simulink model "Vehicle14DOFSystemRack"  (R2024a)
settings: Solver=ode4  StartTime=0.0  StopTime=100  FixedStep=0.001  RelTol=1e-3
values from neighbouring files (symbols this model uses):
  EnvGrvty = 9.81    [Par.m]
  PlntBattChrgMax = 4.493    [Par.m]
  PlntBattNumCellSer = 96    [Par.m]
  PlntBattOpenCirctVolt = [3.17242 3.17242 3.17242 3.17242 3.17242 3.17242 3.17242;3.18272 3.18272 3.18272 3.18272 3.18272 3.18272 3.18272;3.19302 3.19302 3.19302 3.19302 3.19302 3.19302 3.19302;3.20331 3.20331 3.20331 3.20331 3.20331 3.20331 3.20331;3.21361 3.21361 3.21361 3.21361 3.21361 3.21361 3.21361;3.22391 3.22391 3.22391 3.22391 3.22391 3.22391 3.22391;3.23421 3.23421 3.23421 3.23421 3.23421 3.23421 3.23421;3.24451 ...(+5187 chars)    [Par.m]
  PlntBattSocInit = 0.6    [Par.m]
  PlntBattTempBpt = [-40 -30 -20 0 23 45 60]    [Par.m]
  PlntBattTempInitDegC = 25    [Par.m]
  PlntBattVoltSocBpt = [0 0.01 0.02 0.03 0.04 0.05 0.06 0.07 0.08 0.09 0.1 0.11 0.12 0.13 0.14 0.15 0.16 0.17 0.18 0.19 0.2 0.21 0.22 0.23 0.24 0.25 0.26 0.27 0.28 0.29 0.3 0.31 0.32 0.33 0.34 0.35 0.36 0.37 0.38 0.39 0.4 0.41 0.42 0.43 0.44 0.45 0.46 0.47 0.48 0.49 0.5 0.51 0.52 0.53 0.54 0.55 0.56 0.57 0.58 0.59 0.6 0.61 0.62 0.63 0.64 0.65 0.66 0.67 0.68 0.69 0.7 0.71 0.72 0.73 0.74 0.75 0.76 0.77 0.78 0.79 0.8 0.81  ...(+91 chars)    [Par.m]
  PlntDCDCVoltInit = 650    [Par.m]
  PlntDriveshftDamp = 100    [Par.m]
  PlntDriveshftStiff = 500    [Par.m]
  PlntEM1RotDamp = 0.001    [Par.m]
  PlntEM1RotInertia = 0.01    [Par.m]
  PlntEM2RotDamp = 0.001    [Par.m]
  PlntEM2RotInertia = 0.01    [Par.m]
  PlntEM3RotDamp = 0.001    [Par.m]
  PlntEM3RotInertia = 0.01    [Par.m]
  PlntEM4RotDamp = 0.001    [Par.m]
  PlntEM4RotInertia = 0.01    [Par.m]
  PlntEMWhlGearRatioFL = 11.04    [Par.m]
  PlntEMWhlGearRatioFR = 11.04    [Par.m]
  PlntEMWhlGearRatioRL = 11.04    [Par.m]
  PlntEMWhlGearRatioRR = 11.04    [Par.m]
  PlntSteerGearRatio = 52.025    [Par.m]
  PlntVehCGHgtAxl = 0.375    [Par.m]
  PlntVehDstCGFrntAxl = 1.61    [Par.m]
  PlntVehDstCGRearAxl = 1.39    [Par.m]
  PlntVehFrntUnsprgMass = 100    [Par.m]
  PlntVehInitLatPos = 0    [Par.m]
  PlntVehInitLatVel = 0    [Par.m]
  PlntVehInitLongPos = 0    [Par.m]
  PlntVehInitLongVel = 0    [Par.m]
  PlntVehInitPitchAng = 0    [Par.m]
  PlntVehInitPitchRate = 0    [Par.m]
  PlntVehInitRollAng = 0    [Par.m]
  PlntVehInitRollRate = 0    [Par.m]
  PlntVehInitVertPos = 0    [Par.m]
  PlntVehInitVertVel = 0    [Par.m]
  PlntVehInitYawAng = 0    [Par.m]
  PlntVehInitYawRate = 0    [Par.m]
  PlntVehMass = 2497    [Par.m]
  PlntVehPitchMomentInertia = 1922.7    [Par.m]
  PlntVehRearUnsprgMass = 100    [Par.m]
  PlntVehRollMomentInertia = 432.33333333333331    (= 432.333333333)    [Par.m]
  PlntVehTrckWdth = [1.685,1.685]    [Par.m]
  PlntVehYawMomentInertia = 2066    [Par.m]
  PlntWhlNumFrnt = 2    [Par.m]
  PlntWhlNumRear = 2    [Par.m]
  PlntWhlPrsFrnt = 220000    [Par.m]
  PlntWhlPrsRear = 220000    [Par.m]
libraries: autolibsharedcoupling x12, autolibsharedcommon x12, autolibutils x10, autolibmappedmotor x4, autolibcoupling x4, matrix_library x4, vehdynlibsteering x4, vehdynlibsuspension x2, vehdynlibtire x2, vehdynlibtirecommon x2, shared6dof x2, autolibdatasheetbattery x1
(part 1 of 7)
settings Model: Creator=admin  LastModifiedBy=admin

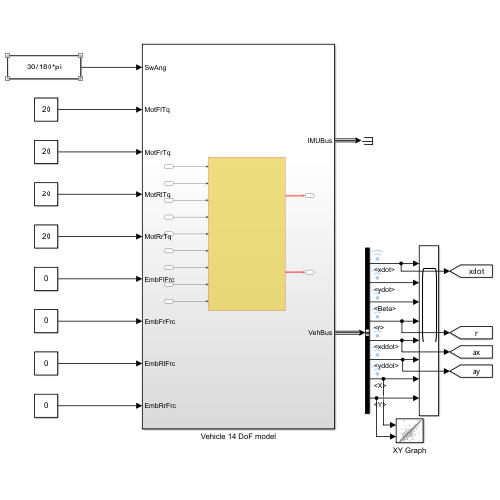
[thumbnail: Simulink's stored preview of the top-level diagram]
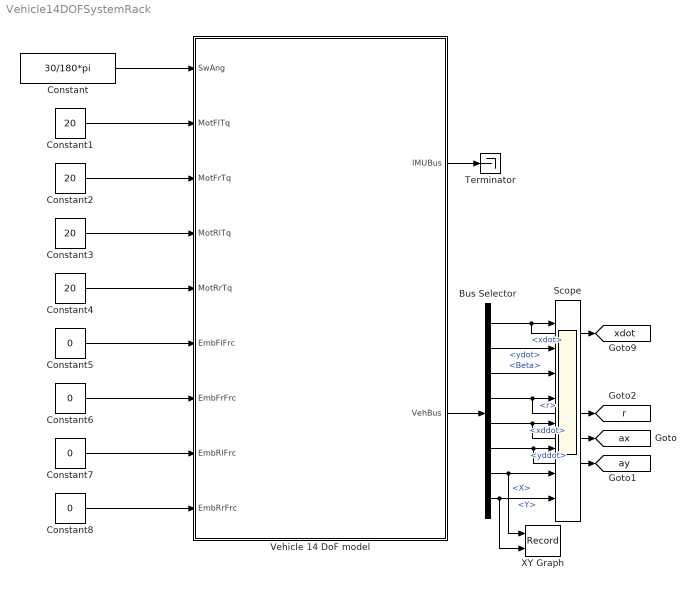
== system Vehicle14DOFSystemRack ==
  Bus Selector : BusSelector  OutputSignals=BdyFrm.Cg.Vel.xdot,BdyFrm.Cg.Vel.ydot,BdyFrm.Cg.Ang.Beta,BdyFrm.Cg.AngVel.r,BdyFrm.Cg.Acc.xddot,BdyFrm.Cg.Acc.yddot,InertFrm.Cg.Disp.X,InertFrm.Cg.Disp.Y
  Constant : Constant  Value=30/180*pi
  Constant{1..4} (4 alike) : Constant  Value=20
  Constant{5..8} (4 alike) : Constant  Value=0
  Scope : Scope  NumInputPorts=8
  Terminator : Terminator
  Vehicle 14 DoF model : Subsystem
  XY Graph : Record  FileSettingsInternal="{\"entries\":[{\"content\":{\"excelSettings\":{\"content\":{},\"type\":\"Streamout.ExcelSettings\"}},\"type\":\"Streamout.FileSettingStorage\",\"uuid\":\"\"}],\"packageUris\":[\"http:\\/\\/schema.mathworks.com\\/mf0\\/streamout_blocks\\/R2020a\"],\"version\":\"1.0\"}"  Layout=[1 1]  SignalsInternal="{\"entries\":[{\"content\":{\"signals\":[{\"content\":{\"blockPath\":[],\"dimensions\":[1],\"domain\":\"\",\"lineColor\":\"#a2142f\",\"plots\":[ 1 ],\"port\":1,\"sid\":[\"\"],\"signalID\":1,\"signalName\":\"<X>\"},\"type\":\"RecordBlkView.Signal\",\"uuid\":\"\"},{\"content\":{\"blockPath\":[],\"dimensions\":[1],\"domain\":\"\",\"lineColor\":\"#139fff\",\"plots\":[ 1 ],\"port\":2,\"sid\":[\"\"],\"signalID\":2,\"signalName\":\"<Y>\"},\"type\":\"RecordBlkView.Signal\",\"uuid\":\"\"}]},\"type\":\"RecordBlkView.InputSignals\",\"uuid\":\"\"}],\"packageUris\":[\"http:\\/\\/schema.mathworks.com\\/mf0\\/streamout_blocks\\/R2020a\"],\"version\":\"1.0\"}"  VisualizationBindings="{\"xyplotplugin\":{\"info\":[{\"series\":[{\"bindingParametersList\":[{\"parameter\":\"X-Axis\",\"signalID\":1,\"signalName\":\"<X>\"},{\"parameter\":\"Y-Axis\",\"signalID\":2,\"signalName\":\"<Y>\"}],\"seriesID\":0}],\"subplotID\":1}]}}"  CompatibilityTag=XY
  tag scope: ax=global, ay=global, r=global, xdot=global
  wires:
  Constant6/1 -> Vehicle 14 DoF model/7(EmbFrFrc)
  Constant5/1 -> Vehicle 14 DoF model/6(EmbFlFrc)
  Constant4/1 -> Vehicle 14 DoF model/5(MotRrTq)
  Constant2/1 -> Vehicle 14 DoF model/3(MotFrTq)
  Constant/1 -> Vehicle 14 DoF model/1(SwAng)
  Constant3/1 -> Vehicle 14 DoF model/4(MotRlTq)
  Constant1/1 -> Vehicle 14 DoF model/2(MotFlTq)
  Constant7/1 -> Vehicle 14 DoF model/8(EmbRlFrc)
  Constant8/1 -> Vehicle 14 DoF model/9(EmbRrFrc)
  Vehicle 14 DoF model/1(IMUBus) -> Terminator/1
  Vehicle 14 DoF model/2(VehBus) -> Bus Selector/1
  Bus Selector/1 -> [xdot], Scope/1  "<xdot>"
  Bus Selector/2 -> Scope/2  "<ydot>"
  Bus Selector/3 -> Scope/3  "<Beta>"
  Bus Selector/4 -> [r], Scope/4  "<r>"
  Bus Selector/5 -> [ax], Scope/5  "<xddot>"
  Bus Selector/7 -> Scope/7, XY Graph/1  "<X>"
  Bus Selector/8 -> Scope/8, XY Graph/2  "<Y>"
  Bus Selector/6 -> [ay], Scope/6  "<yddot>"

== system Vehicle14DOFSystemRack/Vehicle 14 DoF model ==
  SwAng : Inport
  MotFlTq : Inport  Port=2
  MotFrTq : Inport  Port=3
  MotRlTq : Inport  Port=4
  MotRrTq : Inport  Port=5
  EmbFlFrc : Inport  Port=6
  EmbFrFrc : Inport  Port=7
  EmbRlFrc : Inport  Port=8
  EmbRrFrc : Inport  Port=9
  Vehicle 14 DoF model : Subsystem
  IMUBus : Outport
  VehBus : Outport  Port=2
  wires:
  MotRrTq/1 -> Vehicle 14 DoF model/5(MotRrTq)
  MotFrTq/1 -> Vehicle 14 DoF model/3(MotFrTq)
  SwAng/1 -> Vehicle 14 DoF model/1(SwAng)
  MotRlTq/1 -> Vehicle 14 DoF model/4(MotRlTq)
  MotFlTq/1 -> Vehicle 14 DoF model/2(MotFlTq)
  EmbRlFrc/1 -> Vehicle 14 DoF model/8(EmbRlFrc)
  EmbFlFrc/1 -> Vehicle 14 DoF model/6(EmbFlFrc)
  EmbFrFrc/1 -> Vehicle 14 DoF model/7(EmbFrFrc)
  EmbRrFrc/1 -> Vehicle 14 DoF model/9(EmbRrFrc)
  Vehicle 14 DoF model/1(IMUBus) -> IMUBus/1
  Vehicle 14 DoF model/2(VehBus) -> VehBus/1

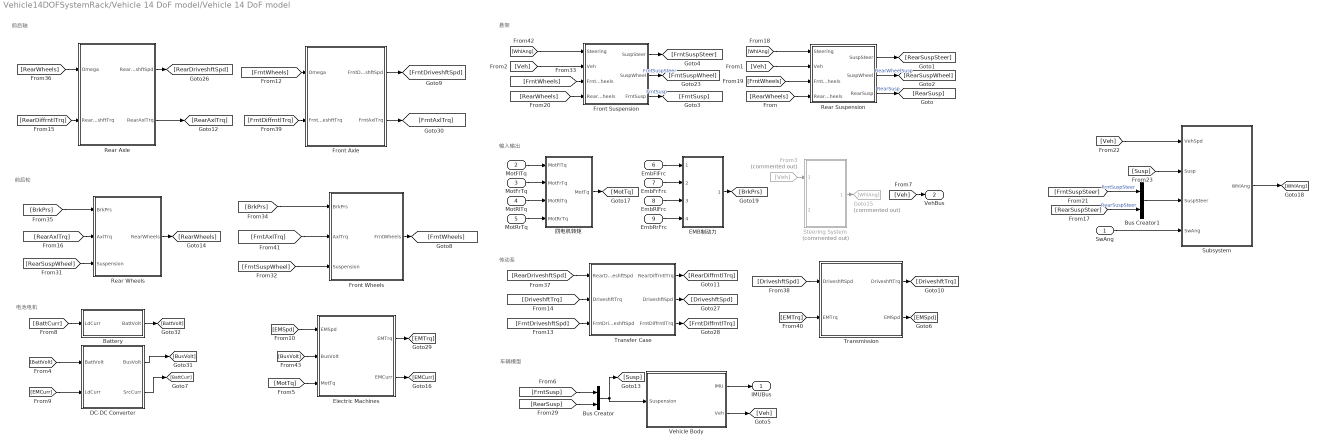
== system Vehicle14DOFSystemRack/Vehicle 14 DoF model/Vehicle 14 DoF model ==
  note: 车辆模型
  note: 传动系
  note: 输入输出
  note: 悬架
  note: 电池电机
  note: 前后轮
  note: 前后轴
  SwAng : Inport
  MotFlTq : Inport  Port=2
  MotFrTq : Inport  Port=3
  MotRlTq : Inport  Port=4
  MotRrTq : Inport  Port=5
  EmbFlFrc : Inport  Port=6
  EmbFrFrc : Inport  Port=7
  EmbRlFrc : Inport  Port=8
  EmbRrFrc : Inport  Port=9
  Battery : Subsystem
  Bus Creator : BusCreator  Inputs=2
  Bus Creator1 : BusCreator  Inputs=2
  DC-DC Converter : Subsystem
  EMB制动力 : Subsystem
  Electric Machines : Subsystem
  From3 : From  Commented=on  GotoTag=Veh
  Front Axle : Subsystem
  Front Suspension : Subsystem
  Front Wheels : Subsystem
  Goto15 : Goto  Commented=on  GotoTag=WhlAng
  Rear Axle : Subsystem
  Rear Suspension : Subsystem
  Rear Wheels : Subsystem
  Steering System : Subsystem  Commented=on
  Subsystem : Subsystem
  Transfer Case : Subsystem
  Transmission : Subsystem
  Vehicle Body : Subsystem
  四电机转矩 : Subsystem
  IMUBus : Outport
  VehBus : Outport  Port=2
  wires:
  EmbRrFrc/1 -> EMB制动力/4(EmbRrFrc)
  [FrntSuspWheel] -> Front Wheels/3(Suspension)
  四电机转矩/1(MotTq) -> [MotTq]
  [FrntDiffrntlTrq] -> Front Axle/2(FrntDriveshftTrq)
  Transmission/2(EMSpd) -> [EMSpd]
  [FrntWheels] -> Rear Suspension/3(FrntWheels)
  MotRlTq/1 -> 四电机转矩/3(MotRlTq)
  EmbFlFrc/1 -> EMB制动力/1(EmbFlFrc)
  [BrkPrs] -> Front Wheels/1(BrkPrs)
  [RearSusp] -> Bus Creator/2
  MotFrTq/1 -> 四电机转矩/2(MotFrTq)
  Electric Machines/1(EMTrq) -> [EMTrq]
  [RearDiffrntlTrq] -> Rear Axle/2(RearDriveshftTrq)
  Front Wheels/1(FrntWheels) -> [FrntWheels]
  Front Suspension/3(FrntSusp) -> [FrntSusp]  "FrntSusp"
  DC-DC Converter/2(SrcCurr) -> [BattCurr]
  [EMTrq] -> Transmission/2(EMTrq)
  [FrntWheels] -> Front Axle/1(Omega)
  [BusVolt] -> Electric Machines/2(BusVolt)
  [WhlAng] -> Rear Suspension/1(Steering)
  Front Suspension/2(SuspWheel) -> [FrntSuspWheel]  "FrntSuspSteer"
  Front Axle/1(FrntDriveshftSpd) -> [FrntDriveshftSpd]
  [BattCurr] -> Battery/1(LdCurr)
  Front Suspension/1(SuspSteer) -> [FrntSuspSteer]
  Vehicle Body/2(Veh) -> [Veh]
  [MotTq] -> Electric Machines/3(MotTq)
  [RearWheels] -> Rear Axle/1(Omega)
  [FrntDriveshftSpd] -> Transfer Case/3(FrntDriveshftSpd)
  Battery/1(BattVolt) -> [BattVolt]
  Rear Axle/2(RearAxlTrq) -> [RearAxlTrq]
  [EMSpd] -> Electric Machines/1(EMSpd)
  [DriveshftSpd] -> Transmission/1(DriveshftSpd)
  From3/1 -> Steering System/1(VehSpd)
  [EMCurr] -> DC-DC Converter/2(LdCurr)
  Rear Wheels/1(RearWheels) -> [RearWheels]
  [RearWheels] -> Rear Suspension/4(RearWheels)
  Bus Creator/1 -> [Susp], Vehicle Body/1(Suspension)
  Transmission/1(DriveshftTrq) -> [DriveshftTrq]
  EmbFrFrc/1 -> EMB制动力/2(EmbFrFrc)
  Rear Suspension/2(SuspWheel) -> [RearSuspWheel]  "RearWheelSusp"
  [BattVolt] -> DC-DC Converter/1(BattVolt)
  [Veh] -> Rear Suspension/2(Veh)
  [DriveshftTrq] -> Transfer Case/2(DriveshftTrq)
  [BrkPrs] -> Rear Wheels/1(BrkPrs)
  MotRrTq/1 -> 四电机转矩/4(MotRrTq)
  Steering System/1(WhlAng) -> Goto15/1
  Rear Suspension/1(SuspSteer) -> [RearSuspSteer]
  Transfer Case/2(DriveshftSpd) -> [DriveshftSpd]
  EMB制动力/1(BrkPrs) -> [BrkPrs]
  MotFlTq/1 -> 四电机转矩/1(MotFlTq)
  [RearDriveshftSpd] -> Transfer Case/1(RearDriveshftSpd)
  Transfer Case/3(FrntDiffrntlTrq) -> [FrntDiffrntlTrq]
  Electric Machines/2(EMCurr) -> [EMCurr]
  Front Axle/2(FrntAxlTrq) -> [FrntAxlTrq]
  [FrntSusp] -> Bus Creator/1
  EmbRlFrc/1 -> EMB制动力/3(EmbRlFrc)
  Rear Suspension/3(RearSusp) -> [RearSusp]  "RearSusp"
  DC-DC Converter/1(BusVolt) -> [BusVolt]
  [RearAxlTrq] -> Rear Wheels/2(AxlTrq)
  [RearSuspWheel] -> Rear Wheels/3(Suspension)
  Rear Axle/1(RearDriveshftSpd) -> [RearDriveshftSpd]
  [FrntAxlTrq] -> Front Wheels/2(AxlTrq)
  Transfer Case/1(RearDiffrntlTrq) -> [RearDiffrntlTrq]
  [Veh] -> Front Suspension/2(Veh)
  [RearWheels] -> Front Suspension/4(RearWheels)
  [FrntWheels] -> Front Suspension/3(FrntWheels)
  [WhlAng] -> Front Suspension/1(Steering)
  Vehicle Body/1(IMU) -> IMUBus/1
  [Veh] -> VehBus/1
  SwAng/1 -> Subsystem/4(SwAng)
  [Veh] -> Subsystem/1(VehSpd)
  Subsystem/1(WhlAng) -> [WhlAng]
  [Susp] -> Subsystem/2(Susp)
  [FrntSuspSteer] -> Bus Creator1/1  "FrntSuspSteer"
  [RearSuspSteer] -> Bus Creator1/2  "RearSuspSteer"
  Bus Creator1/1 -> Subsystem/3(SuspSteer)

== system Vehicle14DOFSystemRack/Vehicle 14 DoF model/Vehicle 14 DoF model/Battery ==
  LdCurr : Inport
  Constant : Constant  Value=27
  Fcn : Fcn  Expr=u+273
  Lithium Ion Battery Pack : autolibdatasheetbattery/Datasheet Battery  CapacityCtrl=Parameter  OutputVlt=Filtered  BattChargeMax=PlntBattChrgMax  Em=interp2(PlntBattTempBpt,PlntBattVoltSocBpt',PlntBattOpenCirctVolt,PlntBattTempInitDegC,PlntBattVoltSocBpt')'  CapLUTBp=PlntBattVoltSocBpt  RInt=PlntBattIntrnRes'  BattTempBp=PlntBattTempBpt+273.15  CapSOCBp=PlntBattSocBpt  Ns=PlntBattNumCellSer  Np=PlntBattNumCellPar  BattCapInit=PlntBattSocInit*PlntBattChrgMax  Tc=PlntBattTimeCnst  Vinit=interp2(PlntBattTempBpt,PlntBattVoltSocBpt,PlntBattOpenCirctVolt*PlntBattNumCellSer,PlntBattTempInitDegC,PlntBattSocInit)  RefBlkName='autolibdatasheetbattery/Datasheet Battery'
  BattVolt : Outport  VectorParamsAs1DForOutWhenUnconnected=off
  wires:
  Lithium Ion Battery Pack/2 -> BattVolt/1
  Constant/1 -> Fcn/1
  Fcn/1 -> Lithium Ion Battery Pack/2
  LdCurr/1 -> Lithium Ion Battery Pack/1  "TotalCurr"

== system Vehicle14DOFSystemRack/Vehicle 14 DoF model/Vehicle 14 DoF model/DC-DC Converter ==
  BattVolt : Inport
  LdCurr : Inport  Port=2
  Bus Selector1 : BusSelector  OutputSignals=PwrLoss  OutputAsBus=on
  Constant3 : Constant  Value=PlntDCDCVoltInit  SampleTime=-1
  Cont LPF : autolibutils/Cont LPF  wc=1  AbsoluteTolerance=auto  aMode=6
  DC-DC Converter : autolibdcdc/Bidirectional DC-DC  Tc=PlntDCDCTimeCnst  Vinit=PlntDCDCVoltInit  Plimit=PlntDCDCPwrLmt  param_loss=Single efficiency measurement  eff=PlntDCDCEff  v_loss_bp=PlntDCDCLossV  i_loss_bp=PlntDCDCLossI  losses_table=PlntDCDCLossTbl  v_eff_bp=[200 400 600 800 1000]  i_eff_bp=[25 50 75 100]  efficiency_table=[96.2 98.1 98.7 99;98.1 99 99.4 99.5;98.7 99.4 99.6 99.7;99 99.5 99.7 99.8;99.2 99.6 99.7 99.8]  x_v_bp=[-1000 -800 -600 -400 -200 200 400 600 800 1000]  x_i_bp=[-100 -75 -50 -25 25 50 75 100]  x_losses_mat=[200.400801603196 225.67703109328 200.803212851408 201.612903225806 199.999999999997 200 225 200;160.320641282556 180.541624874624 201.005025125625 202.020202020203 200 200 180 160;180.541624874624 180.722891566267 181.086519114686 197.568389057748 194.999999999999 179.999999999997 180 180;201.005025125625 181.086519114686 202.020202020203 193.67991845056 190 200 179.999999999997 200;202.020202020203 197.568389057748 193.67991845056 197.505197505197 190 190 194.999999999999 200;200 194.999999999999 190 190 197.505197505197 193.67991845056 197.568389057748 202.020202020203;200 179.999999999997 200 190 193.67991845056 202.020202020203 181.086519114686 201.005025125625;180 180 179.999999999997 194.999999999999 197.568389057748 181.086519114686 180.722891566267 180.541624874624;160 180 200 200 202.020202020203 201.005025125625 180.541624874624 160.320641282556;200 225 200 199.999999999997 201.612903225806 200.803212851408 225.67703109328 200.400801603196]  RefBlkName='autolibdcdc/Bidirectional DC-DC'  CalLossMapData={'BaseCageProjectFileName','';'BaseMbcProjectFileName','';'TaskName','Calibrate Inverter Loss Map';'ChildTasks',{{'DataName','';'TaskName','Import Loss Data'},{'TaskName','Generate Response Models'},{'TaskName','Generate Calibration'},{'TaskName','Update Block Parameters'}}}
  BusVolt : Outport  VectorParamsAs1DForOutWhenUnconnected=off
  SrcCurr : Outport  Port=2  VectorParamsAs1DForOutWhenUnconnected=off
  wires:
  Bus Selector1/1 -> Cont LPF/1
  LdCurr/1 -> DC-DC Converter/3
  BattVolt/1 -> DC-DC Converter/2
  DC-DC Converter/2 -> BusVolt/1
  DC-DC Converter/1 -> Bus Selector1/1
  Constant3/1 -> DC-DC Converter/1
  DC-DC Converter/3 -> SrcCurr/1

== system Vehicle14DOFSystemRack/Vehicle 14 DoF model/Vehicle 14 DoF model/EMB制动力 ==
  EmbFlFrc : Inport
  EmbFrFrc : Inport  Port=2
  EmbRlFrc : Inport  Port=3
  EmbRrFrc : Inport  Port=4
  Bus Creator : BusCreator  Inputs=4
  Gain{1..4} (4 alike) : Gain  Gain=1/(pi*0.145*0.145)
  Transfer Fcn{,1..3} (4 alike) : TransferFcn  Denominator=[0.01 1]
  BrkPrs : Outport
  wires:
  EmbRrFrc/1 -> Gain1/1
  EmbFlFrc/1 -> Gain2/1
  EmbRlFrc/1 -> Gain4/1
  EmbFrFrc/1 -> Gain3/1
  Gain3/1 -> Transfer Fcn2/1
  Gain2/1 -> Transfer Fcn/1
  Transfer Fcn3/1 -> Bus Creator/3
  Gain1/1 -> Transfer Fcn1/1
  Gain4/1 -> Transfer Fcn3/1
  Transfer Fcn/1 -> Bus Creator/1
  Transfer Fcn2/1 -> Bus Creator/2
  Transfer Fcn1/1 -> Bus Creator/4
  Bus Creator/1 -> BrkPrs/1

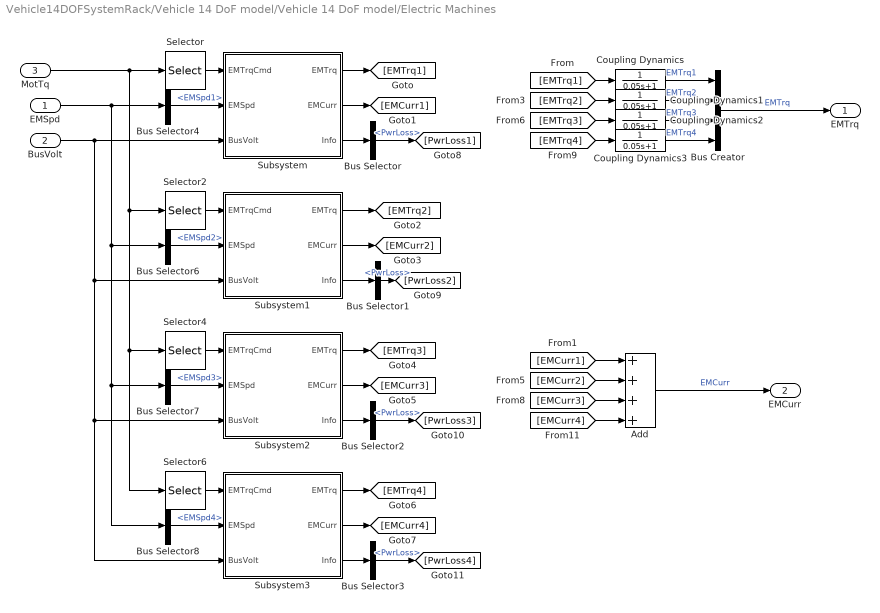
== system Vehicle14DOFSystemRack/Vehicle 14 DoF model/Vehicle 14 DoF model/Electric Machines ==
  EMSpd : Inport
  BusVolt : Inport  Port=2
  MotTq : Inport  Port=3
  Add : Sum  Inputs=++++
  Bus Creator : BusCreator  Inputs=4
  Bus Selector{,1..3} (4 alike) : BusSelector  OutputSignals=PwrLoss
  Bus Selector4 : BusSelector  OutputSignals=EMSpd1
  Bus Selector6 : BusSelector  OutputSignals=EMSpd2
  Bus Selector7 : BusSelector  OutputSignals=EMSpd3
  Bus Selector8 : BusSelector  OutputSignals=EMSpd4
  Coupling Dynamics{,1..3} (4 alike) : TransferFcn  Denominator=[0.05 1]
  Selector : Selector  InputPortWidth=4  IndexOptions=Index vector (dialog)  Indices=[1]  OutputSizes=1
  Selector2 : Selector  InputPortWidth=4  IndexOptions=Index vector (dialog)  Indices=[2]  OutputSizes=1
  Selector4 : Selector  InputPortWidth=4  IndexOptions=Index vector (dialog)  Indices=[3]  OutputSizes=1
  Selector6 : Selector  InputPortWidth=4  IndexOptions=Index vector (dialog)  Indices=[4]  OutputSizes=1
  Subsystem : Subsystem
  Subsystem1 : Subsystem
  Subsystem2 : Subsystem
  Subsystem3 : Subsystem
  EMTrq : Outport
  EMCurr : Outport  Port=2
  wires:
  Bus Selector4/1 -> Subsystem/2(EMSpd)  "<EMSpd1>"
  [EMCurr2] -> Add/2
  Bus Selector1/1 -> [PwrLoss2]  "<PwrLoss>"
  [EMCurr3] -> Add/3
  Subsystem1/3(Info) -> Bus Selector1/1
  Bus Selector3/1 -> [PwrLoss4]  "<PwrLoss>"
  Bus Selector6/1 -> Subsystem1/2(EMSpd)  "<EMSpd2>"
  Subsystem3/1(EMTrq) -> [EMTrq4]
  Subsystem2/3(Info) -> Bus Selector2/1
  Selector2/1 -> Subsystem1/1(EMTrqCmd)
  [EMTrq3] -> Coupling Dynamics2/1
  Selector4/1 -> Subsystem2/1(EMTrqCmd)
  Coupling Dynamics2/1 -> Bus Creator/3  "EMTrq3"
  Bus Selector/1 -> [PwrLoss1]  "<PwrLoss>"
  Subsystem3/3(Info) -> Bus Selector3/1
  Bus Selector2/1 -> [PwrLoss3]  "<PwrLoss>"
  Bus Selector7/1 -> Subsystem2/2(EMSpd)  "<EMSpd3>"
  Subsystem2/1(EMTrq) -> [EMTrq3]
  BusVolt/1 -> Subsystem/3(BusVolt), Subsystem1/3(BusVolt), Subsystem3/3(BusVolt), Subsystem2/3(BusVolt)
  Subsystem1/1(EMTrq) -> [EMTrq2]
  MotTq/1 -> Selector6/1, Selector4/1, Selector2/1, Selector/1
  [EMCurr4] -> Add/4
  [EMTrq4] -> Coupling Dynamics3/1
  Subsystem2/2(EMCurr) -> [EMCurr3]
  Subsystem/3(Info) -> Bus Selector/1
  Coupling Dynamics/1 -> Bus Creator/1  "EMTrq1"
  EMSpd/1 -> Bus Selector4/1, Bus Selector6/1, Bus Selector8/1, Bus Selector7/1
  Selector6/1 -> Subsystem3/1(EMTrqCmd)
  Subsystem/1(EMTrq) -> [EMTrq1]
  Coupling Dynamics3/1 -> Bus Creator/4  "EMTrq4"
  Selector/1 -> Subsystem/1(EMTrqCmd)
  Subsystem/2(EMCurr) -> [EMCurr1]
  Add/1 -> EMCurr/1  "EMCurr"
  [EMTrq1] -> Coupling Dynamics/1
  Bus Creator/1 -> EMTrq/1  "EMTrq"
  [EMCurr1] -> Add/1
  Subsystem1/2(EMCurr) -> [EMCurr2]
  Bus Selector8/1 -> Subsystem3/2(EMSpd)  "<EMSpd4>"
  [EMTrq2] -> Coupling Dynamics1/1
  Subsystem3/2(EMCurr) -> [EMCurr4]
  Coupling Dynamics1/1 -> Bus Creator/2  "EMTrq2"

== system Vehicle14DOFSystemRack/Vehicle 14 DoF model/Vehicle 14 DoF model/Front Axle ==
  Omega : Inport
  FrntDriveshftTrq : Inport  Port=2
  Bus Creator : BusCreator  Inputs=2
  Bus Selector : BusSelector  OutputSignals=Wheels.Omega
  Constant : Constant  Value=[0 0 0 0]
  Demux1 : Demux  Outputs=2
  Front Axle : Subsystem
  Front Axle Compliances : Subsystem
  Selector1 : Selector  InputPortWidth=4  IndexOptions=Index vector (dialog)  Indices=[3 4]  OutputSizes=1
  Subsystem : Subsystem
  FrntDriveshftSpd : Outport
  FrntAxlTrq : Outport  Port=2
  wires:
  Constant/1 -> Selector1/1
  Demux1/1 -> Front Axle/1(Prs1)
  Selector1/1 -> Demux1/1
  Demux1/2 -> Front Axle/2(Prs2)
  FrntDriveshftTrq/1 -> Front Axle/3(DriveshftTrq)
  Front Axle/2(DriveshftSpd) -> FrntDriveshftSpd/1
  Front Axle/3(Axl1Spd) -> Front Axle Compliances/1(RSpdL)
  Front Axle/4(Axl2Spd) -> Front Axle Compliances/2(RSpdR)
  Front Axle Compliances/2(RTrqR) -> Front Axle/5(Axl2Trq)
  Front Axle Compliances/1(RTrqL) -> Front Axle/4(Axl1Trq)
  Bus Selector/1 -> Subsystem/1(Omega)  "<Omega>"
  Omega/1 -> Bus Selector/1
  Subsystem/1(Omega_FL) -> Front Axle Compliances/3(OmegaL)
  Subsystem/2(Omega_FR) -> Front Axle Compliances/4(OmegaR)
  Front Axle Compliances/3(CTrqL) -> Bus Creator/1  "AxlTrqFL"
  Front Axle Compliances/4(CTrqR) -> Bus Creator/2  "AxlTrqFR"
  Bus Creator/1 -> FrntAxlTrq/1

== system Vehicle14DOFSystemRack/Vehicle 14 DoF model/Vehicle 14 DoF model/Front Suspension ==
  Steering : Inport
  Veh : Inport  Port=2
  FrntWheels : Inport  Port=3
  RearWheels : Inport  Port=4
  Bus Creator : BusCreator  Inputs=2
  Bus Selector : BusSelector  OutputSignals=Wheels
  Bus Selector1 : BusSelector  OutputSignals=Wheels
  Kinematics and Compliance Independent Suspension : Subsystem
  Subsystem : Subsystem
  Susp2Wheel : Subsystem
  Wheel2Susp : Subsystem
  Wheel2SuspFrntOnly : Subsystem
  SuspSteer : Outport
  SuspWheel : Outport  Port=2
  FrntSusp : Outport  Port=3
  wires:
  Wheel2SuspFrntOnly/1(Wheels2Susp) -> SuspSteer/1
  FrntWheels/1 -> Bus Selector/1
  Kinematics and Compliance Independent Suspension/2(SuspensionFull) -> Susp2Wheel/1(Susp)
  Susp2Wheel/2(SuspFdbk) -> Wheel2Susp/3(SuspWheel)
  Bus Selector/1 -> Subsystem/1(Frnt), Susp2Wheel/3(Wheels), Wheel2SuspFrntOnly/2(Wheels)  "<Wheels>"
  Veh/1 -> Kinematics and Compliance Independent Suspension/2(Vehicle), Wheel2Susp/1(Veh), Wheel2SuspFrntOnly/1(Veh)
  Bus Creator/1 -> FrntSusp/1  "FrntSusp"
  RearWheels/1 -> Bus Selector1/1
  Subsystem/1(Wheels) -> Wheel2Susp/2(Wheels)
  Wheel2Susp/1(Wheels2Susp) -> Kinematics and Compliance Independent Suspension/3(Wheel), Susp2Wheel/2(WheelSusp)
  Steering/1 -> Kinematics and Compliance Independent Suspension/1(Steering)
  Bus Selector1/1 -> Subsystem/2(Rear)  "<Wheels>"
  Susp2Wheel/1(SuspWheel) -> SuspWheel/1, Bus Creator/2, Wheel2SuspFrntOnly/3(SuspWheel)  "FrntSuspWheel"
  Kinematics and Compliance Independent Suspension/1(Suspension) -> Bus Creator/1  "FrntSuspChassis"

== system Vehicle14DOFSystemRack/Vehicle 14 DoF model/Vehicle 14 DoF model/Front Wheels ==
  BrkPrs : Inport
  AxlTrq : Inport  Port=2
  Suspension : Inport  Port=3
  Add : Sum  Inputs=+-
  Bus Creator1 : BusCreator  Inputs=2
  Bus Creator3 : BusCreator  Inputs=3
  Bus Selector : BusSelector  OutputSignals=Vx,Vy,WhlAng,YawRate,Fext
  Bus Creator : Subsystem
  Bus to Vector : BusToVector
  Clock : Clock
  Constant : Constant  Value=[0.8 0.8 0.8 0.8]
  Constant1 : Constant  Value=[0 0 0 0]
  Constant2 : Constant  Value=repmat(eye(3),1,1,4)
  Constant3 : Constant  Value=10
  Constant4 : Constant  Value=[1.0 1.0 1.0 1.0]
  Front Friction : Subsystem
  Front Ground : Subsystem
  MF Tires Vector : Subsystem  VariantControl=MF Tires Vector
  Reshape : Reshape
  Selector : Selector  NumberOfDimensions=2  InputPortWidth=3  IndexOptions=Index vector (dialog),Select all  Indices=[1],1  OutputSizes=1,1
  Selector1 : Selector  NumberOfDimensions=3  IndexOptions=Index vector (dialog),Index vector (dialog),Index vector (dialog)  Indices=[1 2 3],[1 2 3],[1 2]  OutputSizes=1,1,1
  Selector4 : Selector  InputPortWidth=4  IndexOptions=Index vector (dialog)  Indices=[1 2]  OutputSizes=1
  Subsystem : Subsystem
  Switch : Switch  Criteria=u2 > Threshold  SaturateOnIntegerOverflow=off  InputSameDT=off
  FrntWheels : Outport
  wires:
  Subsystem/2(ScaleFctrs) -> MF Tires Vector/9(ScaleFctrs)
  AxlTrq/1 -> Bus to Vector/1
  Bus to Vector/1 -> MF Tires Vector/2(AxlTrq)
  Selector1/1 -> Bus Creator3/3  "DCM"
  Bus Selector/2 -> MF Tires Vector/4(Vy)  "<Vy>"
  Front Friction/1(y) -> Subsystem/2(lamda_mu_y), Subsystem/1(lamda_mu_x), Bus Creator3/1  "mu"
  Reshape/1 -> MF Tires Vector/5(Camber)
  Subsystem/1(Prs) -> MF Tires Vector/8(Prs)
  Front Ground/1(y) -> MF Tires Vector/10(Gnd), Bus Creator3/2  "z"
  Selector4/1 -> MF Tires Vector/1(BrkPrs)
  Bus Selector/5 -> MF Tires Vector/7(Fext)  "<Fext>"
  Bus Selector/1 -> MF Tires Vector/3(Vx)  "<Vx>"
  Bus Selector/3 -> Selector/1  "<WhlAng>"
  Suspension/1 -> Bus Selector/1
  BrkPrs/1 -> Selector4/1
  Bus Selector/4 -> MF Tires Vector/6(YawRate)  "<YawRate>"
  Selector/1 -> Reshape/1
  Constant1/1 -> Front Ground/1(u)
  Constant2/1 -> Selector1/1
  Bus Creator1/1 -> FrntWheels/1
  Bus Creator/1(Wheels) -> Bus Creator1/1  "Wheels"
  MF Tires Vector/1(Wheels) -> Bus Creator/1(Info)
  Bus Creator3/1 -> Bus Creator1/2  "Gnd"
  Clock/1 -> Add/1
  Constant3/1 -> Add/2
  Add/1 -> Switch/2
  Constant/1 -> Switch/3
  Constant4/1 -> Switch/1
  Switch/1 -> Front Friction/1(u)

== system Vehicle14DOFSystemRack/Vehicle 14 DoF model/Vehicle 14 DoF model/Rear Axle ==
  Omega : Inport
  RearDriveshftTrq : Inport  Port=2
  Bus Creator : BusCreator  Inputs=2
  Bus Selector : BusSelector  OutputSignals=Wheels.Omega
  Constant : Constant  Value=[0 0 0 0]
  Demux1 : Demux  Outputs=2
  Rear Axle : Subsystem
  Selector1 : Selector  InputPortWidth=4  IndexOptions=Index vector (dialog)  Indices=[3 4]  OutputSizes=1
  Subsystem : Subsystem
  Subsystem1 : Subsystem
  Terminator1 : Terminator
  RearDriveshftSpd : Outport
  RearAxlTrq : Outport  Port=2
  wires:
  Subsystem/1(RTrqL) -> Rear Axle/4(Axl1Trq)
  Bus Selector/1 -> Subsystem1/1(Omega)  "<Omega>"
  Omega/1 -> Bus Selector/1
  Demux1/2 -> Rear Axle/2(Prs2)
  Subsystem/2(RTrqR) -> Rear Axle/5(Axl2Trq)
  Selector1/1 -> Demux1/1
  RearDriveshftTrq/1 -> Rear Axle/3(DriveshftTrq)
  Demux1/1 -> Rear Axle/1(Prs1)
  Rear Axle/3(Axl1Spd) -> Subsystem/1(RSpdL)
  Rear Axle/4(Axl2Spd) -> Subsystem/2(RSpdR)
  Subsystem1/1(Omega_RL) -> Subsystem/3(OmegaL)
  Subsystem1/2(Omega_RR) -> Subsystem/4(OmegaR)
  Rear Axle/2(DriveshftSpd) -> RearDriveshftSpd/1
  Bus Creator/1 -> RearAxlTrq/1
  Subsystem/3(CTrqL) -> Bus Creator/1  "AxlTrqRL"
  Subsystem/4(CTrqR) -> Bus Creator/2  "AxlTrqRR"
  Constant/1 -> Selector1/1
  Rear Axle/1(Info) -> Terminator1/1

== system Vehicle14DOFSystemRack/Vehicle 14 DoF model/Vehicle 14 DoF model/Rear Suspension ==
  note: Copyright 2022-2023 The MathWorks, Inc.
  Steering : Inport
  Veh : Inport  Port=2
  FrntWheels : Inport  Port=3
  RearWheels : Inport  Port=4
  Bus Creator : BusCreator  Inputs=2
  Bus Selector : BusSelector  OutputSignals=Wheels
  Bus Selector1 : BusSelector  OutputSignals=Wheels
  Kinematics and Compliance Independent Suspension : Subsystem
  Subsystem : Subsystem
  Susp2Wheel : Subsystem
  Wheel2Susp : Subsystem
  Wheel2SuspRearOnly : Subsystem
  SuspSteer : Outport
  SuspWheel : Outport  Port=2
  RearSusp : Outport  Port=3
  wires:
  Bus Selector1/1 -> Subsystem/2(Rear), Susp2Wheel/3(Wheels), Wheel2SuspRearOnly/2(Wheels)  "<Wheels>"
  Subsystem/1(Wheels) -> Wheel2Susp/2(Wheels)
  Kinematics and Compliance Independent Suspension/2(SuspensionFull) -> Susp2Wheel/1(Susp)
  RearWheels/1 -> Bus Selector1/1
  Susp2Wheel/2(SuspFdbk) -> Wheel2Susp/3(SuspWheel)
  Bus Creator/1 -> RearSusp/1  "RearSusp"
  Steering/1 -> Kinematics and Compliance Independent Suspension/1(Steering)
  Susp2Wheel/1(SuspWheel) -> Wheel2SuspRearOnly/3(SuspWheel), SuspWheel/1, Bus Creator/2  "RearSuspWheel"
  Wheel2SuspRearOnly/1(Wheels2Susp) -> SuspSteer/1
  Wheel2Susp/1(Wheels2Susp) -> Kinematics and Compliance Independent Suspension/3(Wheel), Susp2Wheel/2(WheelSusp)
  Bus Selector/1 -> Subsystem/1(Frnt)  "<Wheels>"
  FrntWheels/1 -> Bus Selector/1
  Kinematics and Compliance Independent Suspension/1(Suspension) -> Bus Creator/1  "RearSuspChassis"
  Veh/1 -> Kinematics and Compliance Independent Suspension/2(Vehicle), Wheel2Susp/1(Veh), Wheel2SuspRearOnly/1(Veh)

== system Vehicle14DOFSystemRack/Vehicle 14 DoF model/Vehicle 14 DoF model/Rear Wheels ==
  BrkPrs : Inport
  AxlTrq : Inport  Port=2
  Suspension : Inport  Port=3
  Add : Sum  Inputs=+-
  Bus Creator1 : BusCreator  Inputs=2
  Bus Creator3 : BusCreator  Inputs=3
  Bus Selector : BusSelector  OutputSignals=Vx,Vy,WhlAng,YawRate,Fext
  Bus Creator : Subsystem
  Bus to Vector : BusToVector
  Clock : Clock
  Constant : Constant  Value=[0.8 0.8 0.8 0.8]
  Constant1 : Constant  Value=[0 0 0 0]
  Constant2 : Constant  Value=repmat(eye(3),1,1,4)
  Constant3 : Constant  Value=10
  Constant4 : Constant  Value=[1.0 1.0 1.0 1.0]
  MF Tires Vector : Subsystem  VariantControl=MF Tires Vector
  Rear Friction : Subsystem
  Rear Ground : Subsystem
  Reshape : Reshape
  Selector : Selector  NumberOfDimensions=2  InputPortWidth=3  IndexOptions=Index vector (dialog),Select all  Indices=[1],1  OutputSizes=1,1
  Selector1 : Selector  NumberOfDimensions=3  IndexOptions=Index vector (dialog),Index vector (dialog),Index vector (dialog)  Indices=[1 2 3],[1 2 3],[3 4]  OutputSizes=1,1,1
  Selector4 : Selector  InputPortWidth=4  IndexOptions=Index vector (dialog)  Indices=[3 4]  OutputSizes=1
  Subsystem : Subsystem
  Switch : Switch  Criteria=u2 > Threshold  SaturateOnIntegerOverflow=off  InputSameDT=off
  RearWheels : Outport  VectorParamsAs1DForOutWhenUnconnected=off
  wires:
  BrkPrs/1 -> Selector4/1
  Rear Friction/1(y) -> Subsystem/2(lamda_mu_y), Subsystem/1(lamda_mu_x), Bus Creator3/1  "mu"
  AxlTrq/1 -> Bus to Vector/1
  Rear Ground/1(y) -> MF Tires Vector/10(Gnd), Bus Creator3/2  "z"
  Selector1/1 -> Bus Creator3/3  "DCM"
  Selector/1 -> Reshape/1
  Bus Selector/4 -> MF Tires Vector/6(YawRate)  "<YawRate>"
  Bus Selector/5 -> MF Tires Vector/7(Fext)  "<Fext>"
  Bus Selector/2 -> MF Tires Vector/4(Vy)  "<Vy>"
  Suspension/1 -> Bus Selector/1
  Bus Selector/3 -> Selector/1  "<WhlAng>"
  Bus Selector/1 -> MF Tires Vector/3(Vx)  "<Vx>"
  Bus to Vector/1 -> MF Tires Vector/2(AxlTrq)
  Selector4/1 -> MF Tires Vector/1(BrkPrs)
  Subsystem/1(Prs) -> MF Tires Vector/8(Prs)
  Subsystem/2(ScaleFctrs) -> MF Tires Vector/9(ScaleFctrs)
  MF Tires Vector/1(Wheels) -> Bus Creator/1(Info)
  Bus Creator/1(Wheels) -> Bus Creator1/1  "Wheels"
  Bus Creator3/1 -> Bus Creator1/2  "Gnd"
  Bus Creator1/1 -> RearWheels/1
  Constant1/1 -> Rear Ground/1(u)
  Constant2/1 -> Selector1/1
  Reshape/1 -> MF Tires Vector/5(Camber)
  Constant/1 -> Switch/3
  Switch/1 -> Rear Friction/1(u)
  Constant3/1 -> Add/2
  Constant4/1 -> Switch/1
  Clock/1 -> Add/1
  Add/1 -> Switch/2

== system Vehicle14DOFSystemRack/Vehicle 14 DoF model/Vehicle 14 DoF model/Steering System ==
  VehSpd : Inport
  SwAng : Inport  Port=2
  Bus Creator1 : BusCreator  Inputs=2
  Bus Creator2 : BusCreator  Inputs=1
  Bus Creator3 : BusCreator  Inputs=2
  Bus Creator4 : BusCreator  Inputs=1
  Bus Creator5 : BusCreator  Inputs=2
  Bus Selector : BusSelector  OutputSignals=BdyFrm.Cg.Vel.xdot
  Bus Selector1 : BusSelector  OutputSignals=Front.WhlAng.FL,Front.WhlAng.FR,Rear.WhlAng.RL,Rear.WhlAng.RR  OutputAsBus=on
  Bus to Vector : BusToVector
  Constant : Constant  Value=0  SampleTime=-1
  Front Steering : vehdynlibsteering/Mapped Steering  SpdDpd=on  IndexType=Rack travel displacement  GrType=Constant  StrgAngBpts=[-1.5*pi 1.5*pi]  RackDispBpts=PlntSteerRackDispBpt  Gr=PlntSteerGearRatio  GrTbl=[9.87 9.87 7.16 7.16 9.87 9.87]*2*pi  WhlLftTbl=PlntSteerLftWhlAngTbl  WhlRghtTbl=PlntSteerRghtWhlAngTbl  VehSpdBpts=[-1 1]  SpdFctTbl=[1 1]  aMode=2
  Rear Steering : vehdynlibsteering/Mapped Steering  SpdDpd=on  IndexType=Rack travel displacement  GrType=Constant  StrgAngBpts=[-1.5*pi 1.5*pi]  RackDispBpts=PlntSteerRackDispBpt  Gr=PlntSteerGearRatio/10  GrTbl=[9.87 9.87 7.16 7.16 9.87 9.87]*2*pi  WhlLftTbl=PlntSteerLftWhlAngTbl  WhlRghtTbl=PlntSteerRghtWhlAngTbl  VehSpdBpts=[-1 1]  SpdFctTbl=[1 1]  aMode=2
  Terminator : Terminator
  Terminator1 : Terminator
  WhlAng : Outport  VectorParamsAs1DForOutWhenUnconnected=off
  wires:
  Rear Steering/1 -> Terminator1/1
  Bus Creator5/1 -> Bus Creator4/1  "WhlAng"
  Front Steering/3 -> Bus Creator3/2  "FR"
  Front Steering/1 -> Terminator/1
  Rear Steering/3 -> Bus Creator5/2  "RR"
  Front Steering/2 -> Bus Creator3/1  "FL"
  Bus Selector/1 -> Rear Steering/2, Front Steering/2  "<xdot>"
  Bus Selector1/1 -> Bus to Vector/1
  Bus Creator3/1 -> Bus Creator2/1  "WhlAng"
  Bus to Vector/1 -> WhlAng/1
  Bus Creator1/1 -> Bus Selector1/1
  Rear Steering/2 -> Bus Creator5/1  "RL"
  VehSpd/1 -> Bus Selector/1
  Bus Creator2/1 -> Bus Creator1/1  "Front"
  Constant/1 -> Rear Steering/1
  Bus Creator4/1 -> Bus Creator1/2  "Rear"
  SwAng/1 -> Front Steering/1

== system Vehicle14DOFSystemRack/Vehicle 14 DoF model/Vehicle 14 DoF model/Subsystem ==
  VehSpd : Inport
  Susp : Inport  Port=2
  SuspSteer : Inport  Port=3
  SwAng : Inport  Port=4
  Bus Creator1 : BusCreator  Inputs=2
  Bus Creator2 : BusCreator  Inputs=1
  Bus Creator3 : BusCreator  Inputs=2
  Bus Creator4 : BusCreator  Inputs=1
  Bus Creator5 : BusCreator  Inputs=2
  Bus Selector : BusSelector  OutputSignals=BdyFrm.Cg.Vel.xdot
  Bus Selector1 : BusSelector  OutputSignals=Front.WhlAng.FL,Front.WhlAng.FR,Rear.WhlAng.RL,Rear.WhlAng.RR  OutputAsBus=on
  Bus Selector2 : BusSelector  OutputSignals=FrntSuspSteer.SuspFrame.Fx,FrntSuspSteer.SuspFrame.Fy,FrntSuspSteer.SuspFrame.Fz,FrntSuspSteer.SuspFrame.Mx,FrntSuspSteer.SuspFrame.My,FrntSuspSteer.SuspFrame.Mz
  Bus Selector3 : BusSelector  OutputSignals=FrntSusp.FrntSuspChassis.Whl.Ang
  Bus Selector4 : BusSelector  OutputSignals=RearSuspSteer.SuspFrame.Fx,RearSuspSteer.SuspFrame.Fy,RearSuspSteer.SuspFrame.Fz,RearSuspSteer.SuspFrame.Mx,RearSuspSteer.SuspFrame.My,RearSuspSteer.SuspFrame.Mz
  Bus Selector5 : BusSelector  OutputSignals=RearSusp.RearSuspChassis.Whl.Ang
  Bus to Vector : BusToVector
  Constant : Constant  Value=0
  Front Steering : vehdynlibsteering/Steering System  StrgType=Rack and pinion  IntmdShaftType=Single Cardan joint  PwrAst=on  AckStr=on  PwrAstOverride=off  AckStrOverride=off  KingpinOverride=off  Loc=Front  StrIn=Angle  TrckWdth=PlntVehTrckWdth(1)  StrRng=PlntSteerRange  DbWdth=0  StrWhlInert=PlntSteerUpperInertia  StrColInert=PlntSteerLowerInertia  KngpnOfst=PlntSteerKngpnOfst  Lambda=PlntSteerLambda  HbLead=PlntSteerHbLead  StcLdRadius=PlntSteerStcLdRadius  OvrlStrRatio=PlntSteerRatio  StrgAngBpts="[-6.2832   -5.0265   -3.7699   -2.5133   -1.2566         0    1.2566    2.5133    3.7699    5.0265    6.2832]"  CstrAng=0  StrgRatioType=Constant  RckGn=PlntSteerRckGn  RckGnTbl=ones(1,11)*0.0057*2*pi  RckPnAlgm=Kinematics  RackDispBpts=[-40 -19.2 -4.53 4.53 19.2 40]  RghtWhlAngTbl=[-1.5*pi -0.72*pi -0.17*pi 0.17*pi 0.72*pi 1.5*pi]/13.5  RghtWhlStrSpdTbl=[0.008726624950158,0.008727065906090,0.008727190569212,0.008727190569212,0.008727065906090,0.008726624950158]  LftWhlAngTbl=[-1.5*pi -0.72*pi -0.17*pi 0.17*pi 0.72*pi 1.5*pi]/13.5  LftWhlStrSpdTbl=[0.008726624950158,0.008727065906090,0.008727190569212,0.008727190569212,0.008727065906090,0.008726624950158]  StrgArmLngth=PlntSteerStrgArmLngth  RckCsLngth=PlntSteerRckCsLngth  TieRodLngth=PlntSteerTieRodLngth  Dst=PlntSteerDst  Epsilon=PlntSteerEpsilon  PnInert=PlntSteerPnInert  SptlAng=2.6178  Alpha_b=2.6178  Alpha_c=2.7051  Sigma_bc=0.2618  Gamma=0.2618  TrqBpts=PlntSteerWheelTrqBpt  VehSpdBpts=[0 20]  TrqTbl=PlntSteerTrqAsstTbl  TrqLmt=PlntSteerTrqLimit  PwrLmt=PlntSteerPwrLimit  Eta=1  omega_c=PlntSteerWc  AckParamType=Constant  PctAck=PlntSteerPctAck  PctAckTbl=ones(1,11)*100  SlgStf=PlntSteerSlgStf  UpprFric=PlntSteerUpprFric  PrsFric=PlntSteerPrsFric  MaxStf=PlntSteerMaxStf  MaxUpprFric=PlntSteerMaxUpprFric  MaxDamp=PlntSteerMaxDamp  TorStf=PlntSteerTorStf  TorDamp=PlntSteerTorDamp  A=0  D=0  I=5  OutSatLowLmt=-500  OutSatUpLmt=500  P=150
  Gain : Gain  Gain=0
  Gain1 : Gain  Gain=0
  Mux : Mux  Inputs=6
  Mux1 : Mux  Inputs=6
  Rear Steering : vehdynlibsteering/Steering System  StrgType=Rack and pinion  IntmdShaftType=Single Cardan joint  PwrAst=on  AckStr=on  PwrAstOverride=off  AckStrOverride=off  KingpinOverride=off  Loc=Rear  StrIn=Angle  TrckWdth=PlntVehTrckWdth(1)  StrRng=PlntSteerRange  DbWdth=0  StrWhlInert=PlntSteerUpperInertia  StrColInert=PlntSteerLowerInertia  KngpnOfst=PlntSteerKngpnOfst  Lambda=PlntSteerLambda  HbLead=PlntSteerHbLead  StcLdRadius=PlntSteerStcLdRadius  OvrlStrRatio=PlntSteerRatio  StrgAngBpts="[-6.2832   -5.0265   -3.7699   -2.5133   -1.2566         0    1.2566    2.5133    3.7699    5.0265    6.2832]"  CstrAng=0  StrgRatioType=Constant  RckGn=PlntSteerRckGn  RckGnTbl=ones(1,11)*0.0057*2*pi  RckPnAlgm=Kinematics  RackDispBpts=[-40 -19.2 -4.53 4.53 19.2 40]  RghtWhlAngTbl=[-1.5*pi -0.72*pi -0.17*pi 0.17*pi 0.72*pi 1.5*pi]/13.5  RghtWhlStrSpdTbl=[0.008726624950158,0.008727065906090,0.008727190569212,0.008727190569212,0.008727065906090,0.008726624950158]  LftWhlAngTbl=[-1.5*pi -0.72*pi -0.17*pi 0.17*pi 0.72*pi 1.5*pi]/13.5  LftWhlStrSpdTbl=[0.008726624950158,0.008727065906090,0.008727190569212,0.008727190569212,0.008727065906090,0.008726624950158]  StrgArmLngth=PlntSteerStrgArmLngth  RckCsLngth=PlntSteerRckCsLngth  TieRodLngth=PlntSteerTieRodLngth  Dst=PlntSteerDst  Epsilon=PlntSteerEpsilon  PnInert=PlntSteerPnInert  SptlAng=2.6178  Alpha_b=2.6178  Alpha_c=2.7051  Sigma_bc=0.2618  Gamma=0.2618  TrqBpts=PlntSteerWheelTrqBpt  VehSpdBpts=[0 20]  TrqTbl=PlntSteerTrqAsstTbl  TrqLmt=PlntSteerTrqLimit  PwrLmt=PlntSteerPwrLimit  Eta=1  omega_c=PlntSteerWc  AckParamType=Constant  PctAck=PlntSteerPctAck  PctAckTbl=ones(1,11)*100  SlgStf=PlntSteerSlgStf  UpprFric=PlntSteerUpprFric  PrsFric=PlntSteerPrsFric  MaxStf=PlntSteerMaxStf  MaxUpprFric=PlntSteerMaxUpprFric  MaxDamp=PlntSteerMaxDamp  TorStf=PlntSteerTorStf  TorDamp=PlntSteerTorDamp  A=0  D=0  I=0  OutSatLowLmt=-500  OutSatUpLmt=500  P=0
  Selector : Selector  NumberOfDimensions=2  InputPortWidth=3  IndexOptions=Index vector (dialog),Index vector (dialog)  Indices=2,[1 2]  OutputSizes=1,1
  Selector1 : Selector  NumberOfDimensions=2  InputPortWidth=3  IndexOptions=Index vector (dialog),Index vector (dialog)  Indices=3,[1 2]  OutputSizes=1,1
  Selector14 : Selector  NumberOfDimensions=2  InputPortWidth=3  IndexOptions=Index vector (dialog),Index vector (dialog)  Indices=2,[1 2]  OutputSizes=1,1
  Selector15 : Selector  NumberOfDimensions=2  InputPortWidth=3  IndexOptions=Index vector (dialog),Index vector (dialog)  Indices=3,[1 2]  OutputSizes=1,1
  Terminator : Terminator
  Terminator1 : Terminator
  WhlAng : Outport  Unit=rad  VectorParamsAs1DForOutWhenUnconnected=off
  wires:
  Selector1/1 -> Front Steering/2
  Mux/1 -> Front Steering/3
  Bus Creator1/1 -> Bus Selector1/1
  Bus to Vector/1 -> WhlAng/1
  VehSpd/1 -> Bus Selector/1
  Bus Creator5/1 -> Bus Creator4/1  "WhlAng"
  Gain1/1 -> Bus Creator5/2  "RR"
  Bus Selector3/1 -> Selector1/1, Selector/1  "<Ang>"
  Rear Steering/1 -> Terminator1/1
  Gain/1 -> Bus Creator5/1  "RL"
  Bus Creator2/1 -> Bus Creator1/1  "Front"
  Front Steering/3 -> Bus Creator3/2  "FR"
  Bus Selector/1 -> Rear Steering/4, Front Steering/4  "<xdot>"
  Rear Steering/3 -> Gain1/1  "RR"
  Front Steering/2 -> Bus Creator3/1  "FL"
  Bus Creator4/1 -> Bus Creator1/2  "Rear"
  Front Steering/1 -> Terminator/1
  Selector/1 -> Front Steering/1
  Bus Selector1/1 -> Bus to Vector/1
  Bus Creator3/1 -> Bus Creator2/1  "WhlAng"
  Rear Steering/2 -> Gain/1  "RL"
  SwAng/1 -> Front Steering/5
  Bus Selector5/1 -> Selector14/1, Selector15/1  "<Ang>"
  Selector15/1 -> Rear Steering/2
  Selector14/1 -> Rear Steering/1
  Susp/1 -> Bus Selector5/1, Bus Selector3/1
  Bus Selector2/1 -> Mux/1  "<Fx>"
  Bus Selector2/5 -> Mux/5  "<My>"
  Bus Selector2/6 -> Mux/6  "<Mz>"
  Bus Selector2/4 -> Mux/4  "<Mx>"
  Bus Selector2/3 -> Mux/3  "<Fz>"
  Bus Selector2/2 -> Mux/2  "<Fy>"
  Constant/1 -> Rear Steering/5
  Bus Selector4/3 -> Mux1/3  "<Fz>"
  Bus Selector4/4 -> Mux1/4  "<Mx>"
  Bus Selector4/5 -> Mux1/5  "<My>"
  Bus Selector4/1 -> Mux1/1  "<Fx>"
  Bus Selector4/6 -> Mux1/6  "<Mz>"
  SuspSteer/1 -> Bus Selector4/1, Bus Selector2/1
  Bus Selector4/2 -> Mux1/2  "<Fy>"
  Mux1/1 -> Rear Steering/3

== system Vehicle14DOFSystemRack/Vehicle 14 DoF model/Vehicle 14 DoF model/Transfer Case ==
  RearDriveshftSpd : Inport
  DriveshftTrq : Inport  Port=2
  FrntDriveshftSpd : Inport  Port=3
  Bus Creator : BusCreator  Inputs=2
  Constant : Constant  Value=0.5  SampleTime=-1
  Constant1 : Constant  Value=0.5  SampleTime=-1
  DriveshftTrq Routing : Subsystem
  Subsystem : Subsystem
  RearDiffrntlTrq : Outport  VectorParamsAs1DForOutWhenUnconnected=off
  DriveshftSpd : Outport  Port=2  VectorParamsAs1DForOutWhenUnconnected=off
  FrntDiffrntlTrq : Outport  Port=3  VectorParamsAs1DForOutWhenUnconnected=off
  wires:
  Constant/1 -> Subsystem/1(TrqSplitRatio)
  Constant1/1 -> Subsystem/2(SpdLock)
  DriveshftTrq/1 -> DriveshftTrq Routing/2(DriveshftTrq)
  Subsystem/3(RearDiffrntlTrq) -> DriveshftTrq Routing/3("TrnsfrCaseRearTrq ")
  Subsystem/2(FrntDiffrntlTrq) -> DriveshftTrq Routing/1(TrnsfrCaseFrntTrq)
  FrntDriveshftSpd/1 -> Bus Creator/1, Subsystem/3(FrntDiffrntlSpd)  "FrntDriveshftSpd"
  DriveshftTrq Routing/2(TrnsfrCaseTrq) -> Subsystem/4(DriveshftTrq)
  DriveshftTrq Routing/3(RearDiffrntlTrq) -> RearDiffrntlTrq/1
  RearDriveshftSpd/1 -> Bus Creator/2, Subsystem/5(RearDiffrntlSpd)  "RearDriveshftSpd"
  Bus Creator/1 -> DriveshftSpd/1
  DriveshftTrq Routing/1(FrntDiffrntlTrq) -> FrntDiffrntlTrq/1

== system Vehicle14DOFSystemRack/Vehicle 14 DoF model/Vehicle 14 DoF model/Transmission ==
  DriveshftSpd : Inport
  EMTrq : Inport  Port=2
  BEV4 : Subsystem
  DriveshftTrq : Outport
  EMSpd : Outport  Port=2
  wires:
  EMTrq/1 -> BEV4/1(EMTrq)
  DriveshftSpd/1 -> BEV4/2(DriveshftSpd)
  BEV4/1(EMSpd) -> EMSpd/1
  BEV4/2(DriveshftTrq) -> DriveshftTrq/1

== system Vehicle14DOFSystemRack/Vehicle 14 DoF model/Vehicle 14 DoF model/Vehicle Body ==
  Suspension : Inport
  Subsystem : Subsystem
  Vehicle 6DOF : Subsystem
  IMU : Outport
  Veh : Outport  Port=2
  wires:
  Suspension/1 -> Vehicle 6DOF/1(Suspension)
  Vehicle 6DOF/1(Veh) -> Veh/1, Subsystem/1(Veh)
  Subsystem/1(IMU) -> IMU/1

== system Vehicle14DOFSystemRack/Vehicle 14 DoF model/Vehicle 14 DoF model/四电机转矩 ==
  MotFlTq : Inport
  MotFrTq : Inport  Port=2
  MotRlTq : Inport  Port=3
  MotRrTq : Inport  Port=4
  Bus Creator : BusCreator  Inputs=4
  MotTq : Outport
  wires:
  MotFlTq/1 -> Bus Creator/1
  MotRlTq/1 -> Bus Creator/3
  MotFrTq/1 -> Bus Creator/2
  Bus Creator/1 -> MotTq/1
  MotRrTq/1 -> Bus Creator/4
